simulink model "scpi_sim_cascade"  (R2024b)
settings: Solver=VariableStepAuto  StartTime=0.0  StopTime=125  RelTol=1e-3
values from neighbouring files (symbols this model uses):
  GT = tf(wn^2,[1 2*wn*zeta wn^2])    [SCPI.m]
  H2 = 0.06/(0.206*s+1)/(0.24*s+1)/(12*s+1)*exp(-0.2*s)    [SCPI.m]
  K = info.SettlingMax/160    [SCPI.m]
  Kr = T/K    [SCPI.m]
  Kr2 = 20.4    [SCPI.m]
  T = info.TransientTime/3    [SCPI.m]
  Td = 0    [SCPI.m]
  Td2 = 0.235    [SCPI.m]
  Ti = T    [SCPI.m]
  Ti2 = 12.24    [SCPI.m]
settings Model: Creator=Student  LastModifiedBy=mihne
settings SolverCC: AlgebraicLoopSolver=TrustRegion
settings DebuggingCC: UnconnectedInputMsg=warning  UnconnectedOutputMsg=warning  UnconnectedLineMsg=warning
settings ModelReferenceCC: EnableRefExpFcnMdlSchedulingChecks=on
settings RTWCC: GPUComputeCapability=3.5  DLArmComputeVersion=19.05

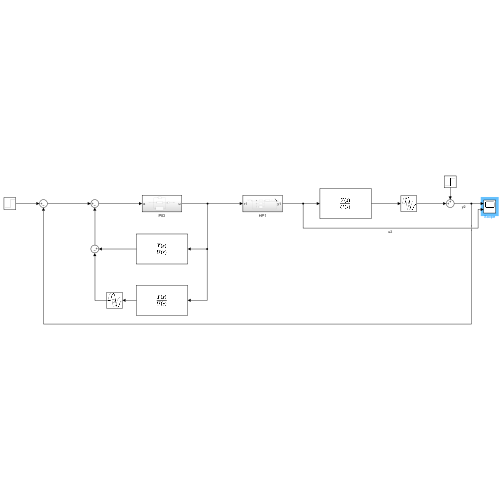
[thumbnail: Simulink's stored preview of the top-level diagram]
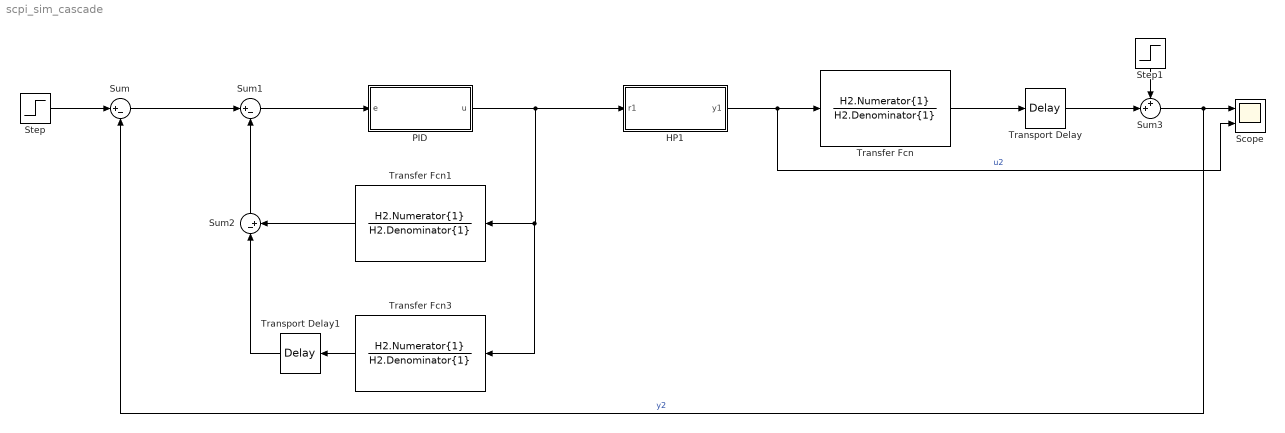
== system scpi_sim_cascade ==
  HP1 : Subsystem
  PID : Subsystem
  Scope : Scope  NumInputPorts=2
  Step : Step  Time=0  After=5  SampleTime=0
  Step1 : Step  Time=75  SampleTime=0
  Sum : Sum  Inputs=|+-
  Sum1 : Sum  Inputs=|+-
  Sum2 : Sum  Inputs=|-+
  Sum3 : Sum  Inputs=++|
  Transfer Fcn : TransferFcn  Numerator=H2.Numerator{1}  Denominator=H2.Denominator{1}
  Transfer Fcn1 : TransferFcn  Numerator=H2.Numerator{1}  Denominator=H2.Denominator{1}
  Transfer Fcn3 : TransferFcn  Numerator=H2.Numerator{1}  Denominator=H2.Denominator{1}
  Transport Delay : TransportDelay  DelayTime=0.2
  Transport Delay1 : TransportDelay  DelayTime=0.2
  wires:
  Step/1 -> Sum/1
  Transport Delay1/1 -> Sum2/1
  Transfer Fcn3/1 -> Transport Delay1/1
  Transfer Fcn/1 -> Transport Delay/1
  Transfer Fcn1/1 -> Sum2/2
  Sum/1 -> Sum1/1
  Sum2/1 -> Sum1/2
  PID/1(u) -> HP1/1(r1), Transfer Fcn3/1, Transfer Fcn1/1
  Sum1/1 -> PID/1(e)
  HP1/1(y1) -> Scope/2, Transfer Fcn/1  "u2"
  Step1/1 -> Sum3/1
  Sum3/1 -> Sum/2, Scope/1  "y2"
  Transport Delay/1 -> Sum3/2

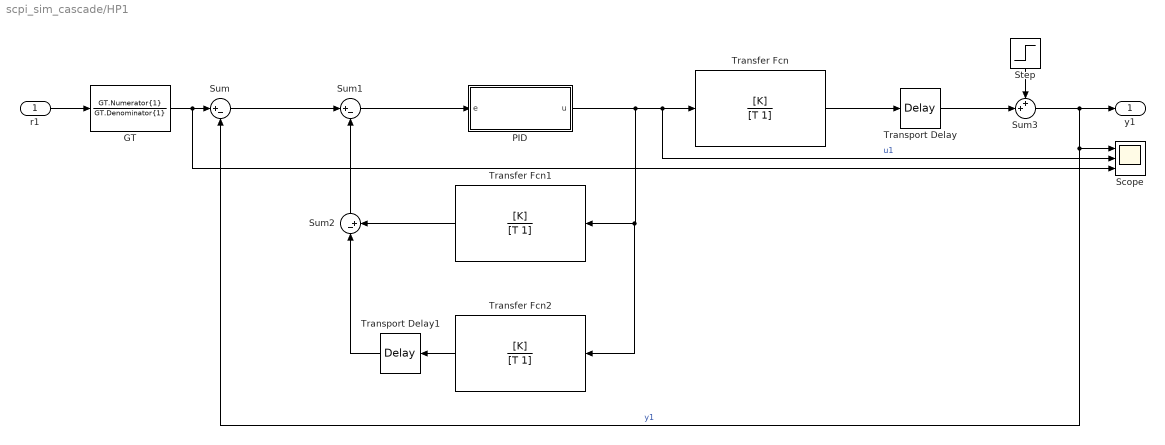
== system scpi_sim_cascade/HP1 ==
  r1 : Inport
  GT : TransferFcn  Numerator=GT.Numerator{1}  Denominator=GT.Denominator{1}
  PID : Subsystem
  Scope : Scope  NumInputPorts=3
  Step : Step  Time=50  After=20  SampleTime=0
  Sum : Sum  Inputs=|+-
  Sum1 : Sum  Inputs=|+-
  Sum2 : Sum  Inputs=|-+
  Sum3 : Sum  Inputs=++|
  Transfer Fcn : TransferFcn  Numerator=[K]  Denominator=[T 1]
  Transfer Fcn1 : TransferFcn  Numerator=[K]  Denominator=[T 1]
  Transfer Fcn2 : TransferFcn  Numerator=[K]  Denominator=[T 1]
  Transport Delay : TransportDelay  DelayTime=0.2
  Transport Delay1 : TransportDelay  DelayTime=0.2
  y1 : Outport
  wires:
  Transfer Fcn1/1 -> Sum2/2
  Transfer Fcn/1 -> Transport Delay/1
  Sum1/1 -> PID/1(e)
  PID/1(u) -> Transfer Fcn2/1, Transfer Fcn1/1, Scope/2, Transfer Fcn/1  "u1"
  Sum/1 -> Sum1/1
  Sum2/1 -> Sum1/2
  Transfer Fcn2/1 -> Transport Delay1/1
  Transport Delay1/1 -> Sum2/1
  Sum3/1 -> Sum/2, Scope/1, y1/1  "y1"
  Step/1 -> Sum3/1
  Transport Delay/1 -> Sum3/2
  r1/1 -> GT/1
  GT/1 -> Scope/3, Sum/1

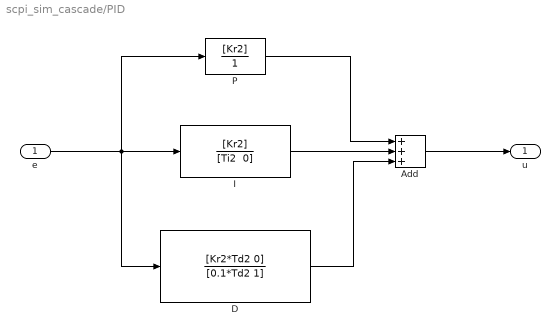
== system scpi_sim_cascade/PID ==
  e : Inport
  Add : Sum  Inputs=+++
  D : TransferFcn  Numerator=[Kr2*Td2 0]  Denominator=[0.1*Td2 1]
  I : TransferFcn  Numerator=[Kr2]  Denominator="[Ti2  0]"
  P : TransferFcn  Numerator=[Kr2]  Denominator=[1]
  u : Outport
  wires:
  e/1 -> P/1, I/1, D/1
  Add/1 -> u/1
  P/1 -> Add/1
  D/1 -> Add/3
  I/1 -> Add/2

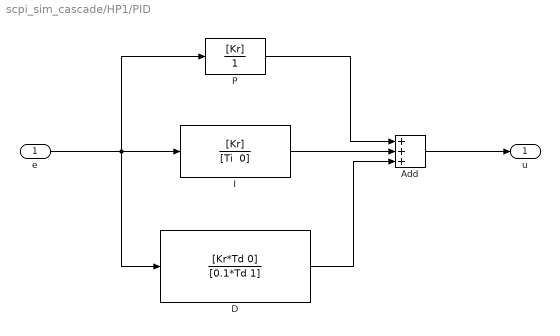
== system scpi_sim_cascade/HP1/PID ==
  e : Inport
  Add : Sum  Inputs=+++
  D : TransferFcn  Numerator=[Kr*Td 0]  Denominator=[0.1*Td 1]
  I : TransferFcn  Numerator=[Kr]  Denominator="[Ti  0]"
  P : TransferFcn  Numerator=[Kr]  Denominator=[1]
  u : Outport
  wires:
  e/1 -> P/1, I/1, D/1
  Add/1 -> u/1
  P/1 -> Add/1
  D/1 -> Add/3
  I/1 -> Add/2
